simulink model "HeatPumpScenario"  (R2022b)
settings: Solver=FixedStepAuto  StartTime=0.0  StopTime=300  FixedStep=1  RelTol=1e-3
PostLoadFcn:
  | load 'sltestHeatpumpBusPostLoadFcn.mat'
  | load 'temp_input.mat'
model workspace (MAT data in the model file):
  Aw = Simulink.Parameter
  Aw.Value = 11.1540749554
  Aw.Description = 'Wall area, 12x10 ft'
  Aw.DataType = 'double'
  Aw.DocUnits = 'm^2'
  Aw.Complexity = 'real'
  Aw.Dimensions = [1 1]
  Lw = Simulink.Parameter
  Lw.Value = 0.177800355601
  Lw.Description = '7 inch wall, expressed in meters'
  Lw.DataType = 'double'
  Lw.DocUnits = 'm'
  Lw.Complexity = 'real'
  Lw.Dimensions = [1 1]
  V = Simulink.Parameter
  V.Value = 40.7932011331
  V.Description = 'Volume of the room (12x12x10ft) converted to m^3'
  V.DataType = 'double'
  V.DocUnits = 'm^3'
  V.Complexity = 'real'
  V.Dimensions = [1 1]
  cpair = Simulink.Parameter
  cpair.Value = 1.004
  cpair.Description = 'specific heat of air, 1.004 kJ/kg-K'
  cpair.DataType = 'double'
  cpair.DocUnits = 'kJ/kg*K'
  cpair.Complexity = 'real'
  cpair.Dimensions = [1 1]
  h = Simulink.Parameter
  h.Value = 25
  h.Description = 'Natural convection coefficient of heat transfer'
  h.DataType = 'double'
  h.DocUnits = 'W/m^2*K'
  h.Complexity = 'real'
  h.Dimensions = [1 1]
  kw = Simulink.Parameter
  kw.Value = 0.67
  kw.Description = 'wall thermal conductivity, assuming a cinderblock wall'
  kw.DataType = 'double'
  kw.DocUnits = 'W/m*K'
  kw.Complexity = 'real'
  kw.Dimensions = [1 1]
  rhoair = Simulink.Parameter
  rhoair.Value = 1.22
  rhoair.Description = 'density of air'
  rhoair.DataType = 'double'
  rhoair.DocUnits = 'kg/m^3'
  rhoair.Complexity = 'real'
  rhoair.Dimensions = [1 1]
undefined symbols (not defined in the file or in its folder): Hecate_Tout, Hecate_Tset
libraries: simulink x1
settings Model: Creator=The MathWorks, Inc.  LastModifiedBy=fedformi_new
settings SolverCC: AlgebraicLoopSolver=TrustRegion
settings DataIOCC: ExternalInput=[t,u]  LimitDataPoints=on  SaveFormat=Array
settings OptimizationCC: LifeSpan=inf
settings DebuggingCC: SolverPrmCheckMsg=warning  UnconnectedInputMsg=warning  UnconnectedOutputMsg=warning  UnconnectedLineMsg=warning  AllowSymbolicDim=off  SFUnexpectedBacktrackingDiag=warning  SFNoUnconditionalDefaultTransitionDiag=warning  SFExecutionAtInitializationDiag=none  SFMachineParentedDataDiag=warning  ArithmeticOperatorsInVariantConditions=warning
settings HardwareCC: ProdBitPerPointer=32  ProdBitPerSizeT=32  ProdBitPerPtrDiffT=32  ProdLargestAtomicFloat=None  ProdIntDivRoundTo=Undefined  ProdEndianess=Unspecified  ProdWordSize=32  ProdHWDeviceType=32-bit Generic
settings ModelReferenceCC: EnableRefExpFcnMdlSchedulingChecks=on  PropagateSignalLabelsOutOfModel=off
settings SFSimCC: SimUseLocalCustomCode=off  CustomCodeUndefinedFunction=UseInterfaceOnly
settings RTWCC: RTWUseLocalCustomCode=off  DLArmComputeVersion=19.05
settings CodeAppCC: StateflowObjectComments=on
settings GRTTargetCC: TargetLangStandard=C89/C90 (ANSI)
settings ConfigComp: CovMetricSettings=dw  CovSaveCumulativeToWorkspaceVar=on  CovSaveSingleToWorkspaceVar=on  CovExternalEMLEnable=off  CovSFcnEnable=off

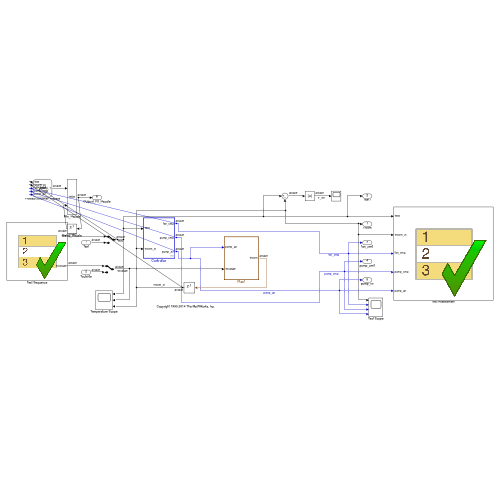
[thumbnail: Simulink's stored preview of the top-level diagram]
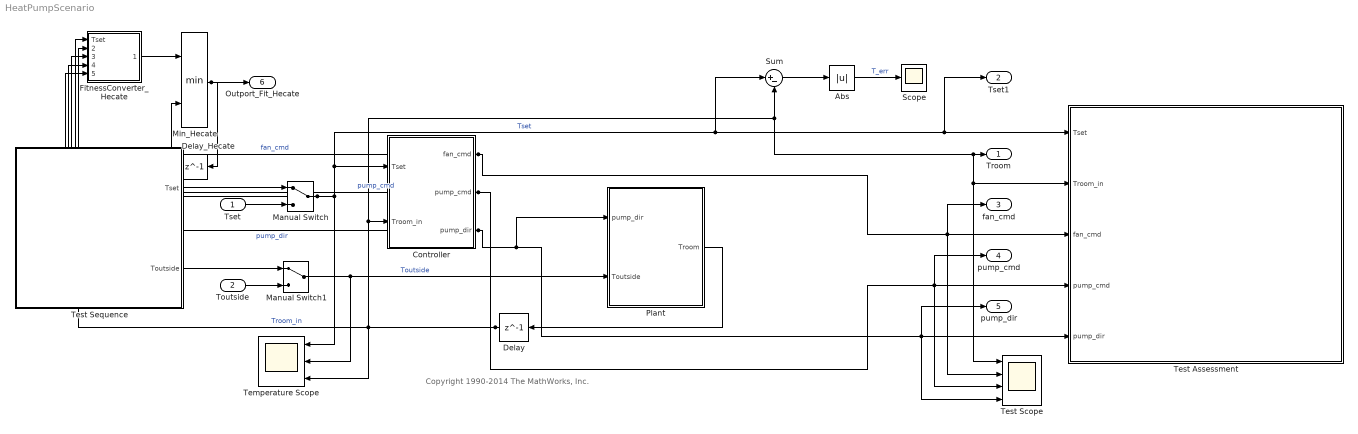
== system HeatPumpScenario ==
  note: Copyright 1990-2014 The MathWorks, Inc.
  Tset : Inport
  Toutside : Inport  Port=2
  Abs : Abs  SaturateOnIntegerOverflow=off
  Controller : Subsystem  TreatAsAtomicUnit=on
  Delay : Delay  DelayLength=1  InitialCondition=75
  Delay_Hecate : Delay  DelayLength=1  InitialCondition=Inf
  FitnessConverter_Hecate : Stateflow chart  TreatAsAtomicUnit=on
  Manual Switch : ManualSwitch
  Manual Switch1 : ManualSwitch
  Min_Hecate : MinMax  Inputs=2
  Plant : Subsystem  TreatAsAtomicUnit=on
      settings: MinAlgLoopOccurrences=on
  Scope : Scope
  Sum : Sum  Inputs=|+-
  Temperature Scope : Scope  NumInputPorts=3
  Test Assessment : Test Sequence  Tag=__SLT_ASMT__  TreatAsAtomicUnit=on
  Test Scope : Scope  NumInputPorts=4
  Test Sequence : Test Sequence  TreatAsAtomicUnit=on
  Troom : Outport
  Tset1 : Outport  Port=2
  fan_cmd : Outport  Port=3
  pump_cmd : Outport  Port=4
  pump_dir : Outport  Port=5
  Outport_Fit_Hecate : Outport  Port=6
  wires:
  Plant/1(Troom) -> Delay/1
  Delay/1 -> Test Scope/1, Test Assessment/2(Troom_in), Troom/1, Sum/2, Controller/2(Troom_in), Temperature Scope/3, FitnessConverter_Hecate/2(Troom_in)  "Troom_in"
  Manual Switch1/1 -> Temperature Scope/2, Plant/2(Toutside)  "Toutside"
  Manual Switch/1 -> Tset1/1, Test Assessment/1(Tset), Sum/1, Controller/1(Tset), Temperature Scope/1, FitnessConverter_Hecate/1(Tset)  "Tset"
  Test Sequence/1(Tset) -> Manual Switch/1
  Test Sequence/2(Toutside) -> Manual Switch1/1
  Toutside/1 -> Manual Switch1/2
  Tset/1 -> Manual Switch/2
  Controller/1(fan_cmd) -> Test Scope/2, Test Assessment/3(fan_cmd), fan_cmd/1, FitnessConverter_Hecate/3(fan_cmd)  "fan_cmd"
  Controller/2(pump_cmd) -> Test Scope/3, Test Assessment/4(pump_cmd), pump_cmd/1, FitnessConverter_Hecate/4(pump_cmd)  "pump_cmd"
  Controller/3(pump_dir) -> Test Scope/4, Test Assessment/5(pump_dir), pump_dir/1, Plant/1(pump_dir), FitnessConverter_Hecate/5(pump_dir)  "pump_dir"
  Sum/1 -> Abs/1
  Abs/1 -> Scope/1  "T_err"
  FitnessConverter_Hecate/1(fitness_1) -> Min_Hecate/1
  Min_Hecate/1 -> Delay_Hecate/1, Outport_Fit_Hecate/1
  Delay_Hecate/1 -> Min_Hecate/2

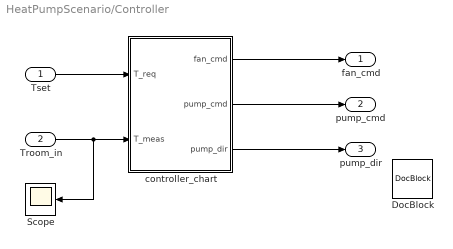
== system HeatPumpScenario/Controller ==
  Tset : Inport
  Troom_in : Inport  Port=2
  DocBlock : simulink/Model-Wide Utilities/DocBlock  DocumentType=Text
      content=|
      | Requirements for the basic Heatpump Controller
      |
      | Temperature difference is defined as the difference between the room and
      | the set temperature.  The controller shall turn the fan on when the
      | temperature difference has reached a certain level, to circulate the air.
      | The controller shall turn the heatpump on when the temperature difference
      | has reached another level, to heat or cool the space.
      |
      | 1. If the temperature difference is less than 2 degrees, the system shall
      | be idle with all signals off.
      | 2. The fan shall activate when the temperature difference is greater than
      | or equal to 2 degrees.
      | 3. The pump shall activate when the temperature difference is greater than
      | or equal to 4 degrees.
      |     3a. If the room temperature is greater than the set temperature, the
      |         system shall cool the space.
      |     3b. If the room temperature is less than the set temperature, the system
      |         shall heat the space.
  Scope : Scope
  controller_chart : Stateflow chart  TreatAsAtomicUnit=on
  fan_cmd : Outport
  pump_cmd : Outport  Port=2
  pump_dir : Outport  Port=3
  wires:
  controller_chart/1(fan_cmd) -> fan_cmd/1
  controller_chart/3(pump_dir) -> pump_dir/1
  controller_chart/2(pump_cmd) -> pump_cmd/1
  Tset/1 -> controller_chart/1(T_req)
  Troom_in/1 -> Scope/1, controller_chart/2(T_meas)

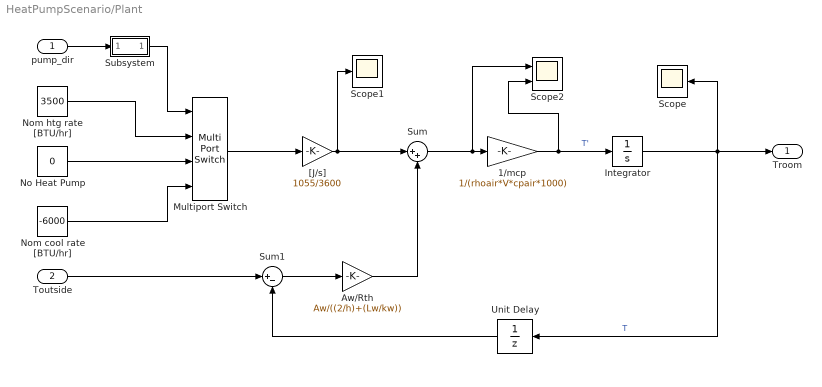
== system HeatPumpScenario/Plant ==
  pump_dir : Inport
  Toutside : Inport  Port=2
  1/mcp : Gain  Gain=1/(rhoair*V*cpair*1000)
  Aw/Rth : Gain  Gain=Aw/((2/h)+(Lw/kw))
  Integrator : Integrator  InitialCondition=75
  Multiport Switch : MultiPortSwitch  SaturateOnIntegerOverflow=off  InputSameDT=off
  No Heat Pump : Constant  Value=0
  Nom cool rate [BTU/hr] : Constant  Value=-6000
  Nom htg rate [BTU/hr] : Constant  Value=3500
  Scope : Scope
  Scope1 : Scope
  Scope2 : Scope  NumInputPorts=2
  Subsystem : Subsystem
  Sum : Sum  Inputs=|++
  Sum1 : Sum  Inputs=|+-
  Unit Delay : UnitDelay  InitialCondition=75  SampleTime=-1  HasFrameUpgradeWarning=on
  "[J/s]" : Gain  Gain=1055/3600
  Troom : Outport
  wires:
  Integrator/1 -> Scope/1, Troom/1, Unit Delay/1  "T"
  Toutside/1 -> Sum1/1
  Nom cool rate [BTU/hr]/1 -> Multiport Switch/4
  Nom htg rate [BTU/hr]/1 -> Multiport Switch/2
  Multiport Switch/1 -> "[J/s]"/1
  Unit Delay/1 -> Sum1/2
  Sum1/1 -> Aw/Rth/1
  Aw/Rth/1 -> Sum/2
  1/mcp/1 -> Scope2/2, Integrator/1  "T'"
  Sum/1 -> Scope2/1, 1/mcp/1
  "[J/s]"/1 -> Sum/1, Scope1/1
  No Heat Pump/1 -> Multiport Switch/3
  pump_dir/1 -> Subsystem/1(In1)
  Subsystem/1(Out1) -> Multiport Switch/1

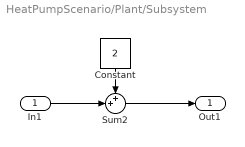
== system HeatPumpScenario/Plant/Subsystem ==
  In1 : Inport
  Constant : Constant  Value=2
  Sum2 : Sum  Inputs=++|
  Out1 : Outport
  wires:
  Sum2/1 -> Out1/1
  In1/1 -> Sum2/2
  Constant/1 -> Sum2/1

== stateflow chart HeatPumpScenario/Test Assessment ==
  state Complete
    state Test_Assessments
      state Check_idle
        %verify(fan_cmd == 0 && pump_cmd == 0 && pump_dir == 0,'All signals must be off at idle');
      state Check_fan
        %verify(fan_cmd == 1 && pump_cmd == 0 && pump_dir == 0, 'Only fan shall be active when 2 < delta T < 4');
      state Else
      (default) -> (junction 81)
      Test_Assessments -> (junction 81)
      (junction 81) -> (junction 82) [order 1] : [abs(Troom_in - Tset) < 2
          | ]
      (junction 82) -> Complete.Test_Assessments.Check_idle [order 1] : [~in(Complete.Test_Assessments.Check_idle)]
      (junction 81) -> (junction 91) [order 2]
      (junction 82) -> (junction 85) [order 2]
      (junction 91) -> (junction 92) [order 1] : [abs(Troom_in - Tset) >= 2 && abs(Troom_in - Tset) < 4
          | ]
      (junction 92) -> Check_fan [order 1] : [~in(Complete.Test_Assessments.Check_fan)]
      (junction 91) -> (junction 100) [order 2]
      (junction 92) -> (junction 95) [order 2]
      (junction 100) -> (junction 101)
      (junction 101) -> Complete.Test_Assessments.Else [order 1] : [~in(Complete.Test_Assessments.Else)]
      (junction 101) -> (junction 104) [order 2]
    (default) -> Test_Assessments
  state Partial
    state step_1
      state Check_idle
        state Check_idle_1
        state Check_idle_2
          verify(fan_cmd >= 0.5 && pump_cmd >= 0.5 && pump_dir >= 0.5);
        (default) -> Check_idle_1
        Check_idle_1 -> Check_idle_2 : [
            | et >= 1
            | ]
      state Else
      (default) -> (junction 121)
      step_1 -> (junction 121)
      (junction 121) -> (junction 122) [order 1] : [Tset <= Troom_in-4 && t >= 10
          | ]
      (junction 122) -> Partial.step_1.Check_idle [order 1] : [~in(Partial.step_1.Check_idle)]
      (junction 121) -> (junction 131) [order 2]
      (junction 122) -> (junction 125) [order 2]
      (junction 131) -> (junction 132)
      (junction 132) -> Partial.step_1.Else [order 1] : [~in(Partial.step_1.Else)]
      (junction 132) -> (junction 135) [order 2]
    (default) -> step_1
  (default) -> Complete [order 1] : [Active_Scenario_Index == 1]
  (default) -> Partial [order 2] : {assert(Active_Scenario_Index == 2,'The value of Scenario Parameter ''Active_Scenario_Index'' is not valid. Use the index of the scenario to specify it.')}
  data: Tset input; Troom_in input; Active_Scenario_Index parameter =2; fan_cmd input; pump_cmd input; pump_dir input

== stateflow chart HeatPumpScenario/Controller/controller_chart ==
  state IDLE
    entry:
    fan_cmd = 0;
    pump_cmd = 0;
    pump_dir = 0;
  state RUNNING
    state IDLE_EXIT
      entry:
      fan_cmd = 0;
      pump_cmd = 0;
      pump_dir = 0;
    state FAN_ONLY
      entry:
      fan_cmd = 1;
      pump_cmd = 0;
      pump_dir = 0;
    state COOLING
      entry:
      fan_cmd = 1;
      pump_cmd = 1;
      pump_dir = 1;
    state HEATING
      entry:
      fan_cmd = 1;
      pump_cmd = 1;
      pump_dir = -1;
    (default) -> FAN_ONLY
    IDLE_EXIT -> FAN_ONLY
    HEATING -> FAN_ONLY : [T_meas > T_req-4]
    COOLING -> FAN_ONLY [order 1] : [T_meas < T_req+4]
    COOLING -> IDLE_EXIT [order 2] : [after(60,sec)]
    FAN_ONLY -> (junction 49) : [mag_T(T_req,T_meas) >= 4]
    (junction 49) -> COOLING [order 1] : [sign_T(T_req, T_meas) == -1]
    (junction 49) -> HEATING [order 2]
  (default) -> IDLE
  RUNNING -> IDLE : [mag_T(T_req,T_meas) <= 2]
  IDLE -> RUNNING : [mag_T(T_req,T_meas) > 2]
  data: T_req_in function_input double size=1; T_meas_in function_input double size=1; Mag function_output double size=1; T_req_in function_input double size=1; T_meas_in function_input double size=1; Tdir function_output double size=1; fan_cmd output double =false; pump_cmd output double =false; pump_dir output double [-1..1] =0; T_req input double size=1; T_meas input double size=1; exit local double =0
  function Mag  = mag_T(T_req_in, T_meas_in):
    | function Mag  = mag_T(T_req_in, T_meas_in)
    | %#codegen
    | 
    | Mag = abs(T_req_in - T_meas_in);
  function Tdir = sign_T(T_req_in,T_meas_in):
    | function Tdir = sign_T(T_req_in,T_meas_in)
    |  %#codegen
    |  
    | Tdir = sign(T_req_in - T_meas_in);

== stateflow chart HeatPumpScenario/FitnessConverter_Hecate ==
  state step_1
    fitness_1 = Inf;
    state Check_idle
      fitness_1 = Inf;
      state Check_idle_1
        fitness_1 = Inf;
      state Check_idle_2
        fitness_1 = min([fan_cmd-(0.5);pump_cmd-(0.5);pump_dir-(0.5);]);
      (default) -> Check_idle_1
      Check_idle_1 -> Check_idle_2 : [et >= 1]
    state Else
      fitness_1 = Inf;
    (default) -> (junction 4)
    Else -> (junction 4) : [(Tset <= Troom_in-4 && t >= 10)]
    (junction 4) -> Check_idle [order 1] : [Tset <= Troom_in-4 && t >= 10]
    (junction 4) -> Else [order 2] : []
    Check_idle -> (junction 4) : [~(Tset <= Troom_in-4 && t >= 10)]
  (default) -> step_1
  data: Tset input; Troom_in input; fan_cmd input; pump_cmd input; pump_dir input; fitness_1 output

== stateflow chart HeatPumpScenario/Test Sequence ==
  state Initialize
    Tset = Hecate_Tset;
    Toutside = Hecate_Tout;
  (default) -> Initialize
  data: Tset output; Toutside output; Hecate_Tset parameter; Hecate_Tout parameter
